simulink model "exp3_heat_storage"  (R2023b)
settings: Solver=VariableStepAuto  StartTime=0.0  StopTime=10.0  RelTol=1e-3
settings Model: Creator=user  LastModifiedBy=user

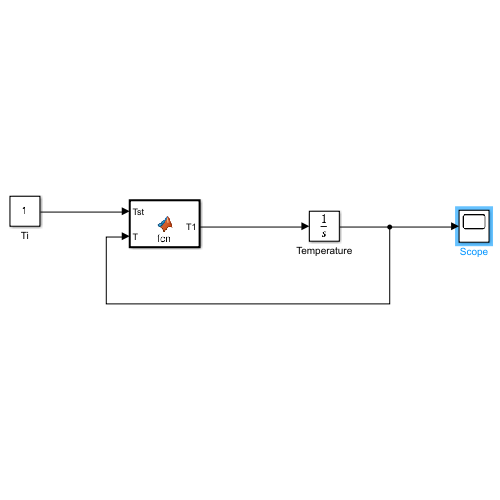
[thumbnail: Simulink's stored preview of the top-level diagram]
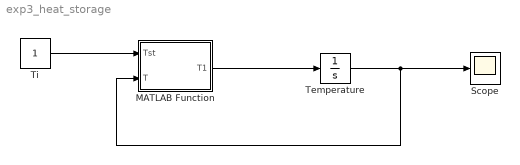
== system exp3_heat_storage ==
  MATLAB Function : MATLAB Function  TreatAsAtomicUnit=on
  Scope : Scope
  Temperature : Integrator
  Ti : Constant
  wires:
  MATLAB Function/1(T1) -> Temperature/1
  Ti/1 -> MATLAB Function/1(Tst)
  Temperature/1 -> MATLAB Function/2(T), Scope/1

== matlab function exp3_heat_storage/MATLAB Function ==
  data: Tst input; T1 output; T input
function T1 = fcn(Tst,T)
V=1;
pho= 1;
At=1;
Cp=1;
U=1;
T1=U*At*(Tst-T)/(V*pho*Cp);
